simulink model "uz_9ph_pmsm_model"  (R2021a)
settings: Solver=FixedStepAuto  StartTime=0.0  StopTime=.5  RelTol=1e-3
PreLoadFcn:
  | uz_pmsm_model_init_parameter
values from neighbouring files (symbols this model uses):
  c = 2/9*cat(1,tl1,tl2,tl3,tl4,tl5,tl6,tl7,tl8,tl9)    [uz_pmsm_model_9ph_init_parameter.m]
  friction_coefficient = 0.001    [uz_pmsm_model_9ph_init_parameter.m]
  inertia = 0.001    [uz_pmsm_model_9ph_init_parameter.m]
  k_i_d = 1000    [uz_pmsm_model_9ph_init_parameter.m]
  k_p_d = 100    [uz_pmsm_model_9ph_init_parameter.m]
  k_p_q = 100    [uz_pmsm_model_9ph_init_parameter.m]
  L_d = 30e-3    (= 0.03)    [uz_pmsm_model_9ph_init_parameter.m]
  L_o1 = 0.01    [uz_pmsm_model_9ph_init_parameter.m]
  L_o2 = 0.01    [uz_pmsm_model_9ph_init_parameter.m]
  L_q = 50e-3    (= 0.05)    [uz_pmsm_model_9ph_init_parameter.m]
  L_x1 = 0.01    [uz_pmsm_model_9ph_init_parameter.m]
  L_x2 = 0.01    [uz_pmsm_model_9ph_init_parameter.m]
  L_y1 = 0.01    [uz_pmsm_model_9ph_init_parameter.m]
  L_y2 = 0.01    [uz_pmsm_model_9ph_init_parameter.m]
  L_zero = 0.01    [uz_pmsm_model_9ph_init_parameter.m]
  polepair = 5    [uz_pmsm_model_9ph_init_parameter.m]
  psi_pm = 0.05    [uz_pmsm_model_9ph_init_parameter.m]
  R_1 = 0.1    [uz_pmsm_model_9ph_init_parameter.m]
  static_friction_torque = 0.01    [uz_pmsm_model_9ph_init_parameter.m]
  ts = 1/1e6    (= 1e-06)    [uz_pmsm_model_9ph_init_parameter.m]
libraries: pid_lib x2
settings Model: DataTypeOverride=Off  Creator=ts  LastModifiedBy=valen
settings SolverCC: AlgebraicLoopSolver=TrustRegion  AutoInsertRateTranBlk=on
settings DataIOCC: LimitDataPoints=on  SaveOutput=off  SaveTime=off
settings OptimizationCC: BlockReduction=off  ConditionallyExecuteInputs=off  DefaultParameterBehavior=Inlined  LifeSpan=inf
settings DebuggingCC: AlgebraicLoopMsg=error  SingleTaskRateTransMsg=error  AllowSymbolicDim=off  StrictBusMsg=ErrorOnBusTreatedAsVector  SFUnexpectedBacktrackingDiag=warning  SFNoUnconditionalDefaultTransitionDiag=warning  SFExecutionAtInitializationDiag=none  SFMachineParentedDataDiag=warning  ArithmeticOperatorsInVariantConditions=warning
settings HardwareCC: ProdBitPerPointer=32  ProdBitPerSizeT=32  ProdBitPerPtrDiffT=32  ProdLargestAtomicFloat=None  ProdIntDivRoundTo=Undefined  ProdEndianess=Unspecified  ProdWordSize=32  ProdHWDeviceType=ASIC/FPGA->ASIC/FPGA  ProdEqTarget=off
settings SFSimCC: SimUseLocalCustomCode=off  CustomCodeUndefinedFunction=UseInterfaceOnly
settings RTWCC: RTWUseLocalCustomCode=off
settings CodeAppCC: StateflowObjectComments=on
settings GRTTargetCC: TargetLangStandard=C89/C90 (ANSI)
settings ConfigComp: CovScope=ReferencedModels  CovMetricSettings=dw  CovSaveCumulativeToWorkspaceVar=on  CovSaveSingleToWorkspaceVar=on  CovExternalEMLEnable=off  CovSFcnEnable=off

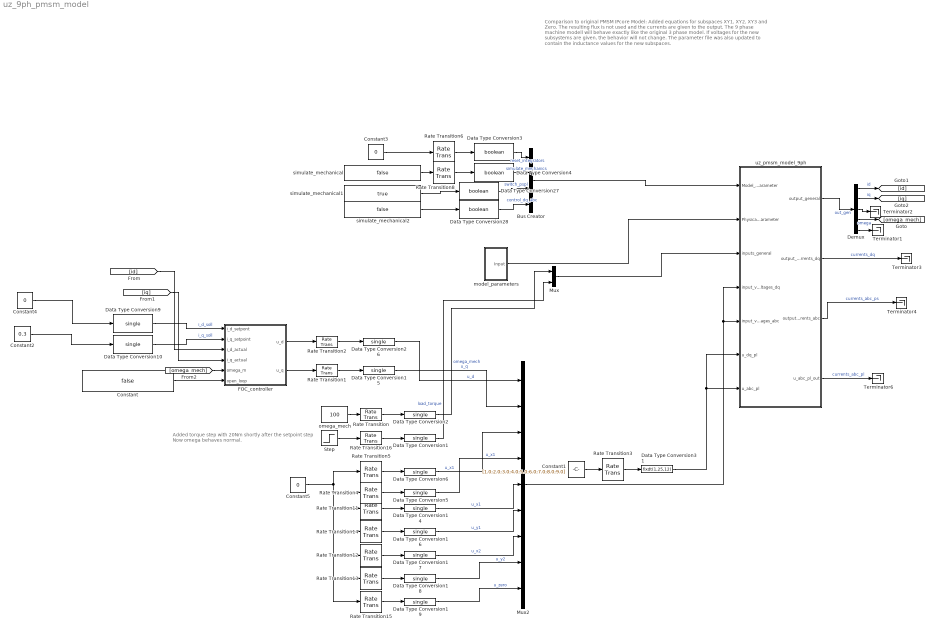
== system uz_9ph_pmsm_model ==
  note: Added torque step with 20Nm shortly after the setpoint step
      | Now omega behaves normal.
  note: Comparison to original PMSM IPcore Model:
      | Added equations for subspaces XY1, XY2, XY3 and Zero. The resulting flux is not used and the currents are given to the output.
      | The 9 phase machine modell will behave exactly like the original 3 phase model. If voltages for the new subsystems are given, the behavior will not change.
      | The parameter file was also updated to contain the inductance values for the new subspaces.
  Bus Creator : BusCreator  Inputs=4
  Constant : Constant  Value=false
  Constant1 : Constant  Value=[1.0;2.0;3.0;4.0;5.0;6.0;7.0;8.0;9.0]
  Constant2 : Constant  Value=0.3
  Constant3 : Constant  Value=0
  Constant4 : Constant  Value=0
  Constant5 : Constant  Value=0
  Data Type Conversion{1..2,5..6,14..19,26} (11 alike) : DataTypeConversion  OutDataTypeStr=single  RndMeth=Nearest
  Data Type Conversion10 : DataTypeConversion  OutDataTypeStr=single
  Data Type Conversion{3..4,27..28} (4 alike) : DataTypeConversion  OutDataTypeStr=boolean
  Data Type Conversion31 : DataTypeConversion  OutDataTypeStr=fixdt(1,25,12)  RndMeth=Nearest
  Data Type Conversion9 : DataTypeConversion  OutDataTypeStr=single
  Demux : Demux  Outputs=5
  FOC_controller : Subsystem
  Mux : Mux  Inputs=2
  Mux2 : Mux  Inputs=9
  Rate Transition{,1..6,8,11..16} (14 alike) : RateTransition  OutPortSampleTime=ts
  Step : Step  Time=0.25  After=20  SampleTime=0
  Terminator{1..4,6} (5 alike) : Terminator
  model_parameters : Subsystem
  omega_mech : Constant  Value=100
  simulate_mechanical : Constant  Value=false
  simulate_mechanical1 : Constant  Value=true
  simulate_mechanical2 : Constant  Value=false
  uz_pmsm_model_9ph : Subsystem  TreatAsAtomicUnit=on
  wires:
  Rate Transition/1 -> Data Type Conversion2/1
  Rate Transition1/1 -> Data Type Conversion15/1
  Rate Transition2/1 -> Data Type Conversion26/1
  Rate Transition6/1 -> Data Type Conversion3/1
  Constant3/1 -> Rate Transition6/1
  Rate Transition8/1 -> Data Type Conversion4/1
  simulate_mechanical/1 -> Rate Transition8/1
  Step/1 -> Rate Transition16/1
  Rate Transition16/1 -> Data Type Conversion1/1
  Constant4/1 -> Data Type Conversion9/1
  uz_pmsm_model_9ph/1(output_general) -> Demux/1  "out_gen"
  Data Type Conversion9/1 -> FOC_controller/1(i_d_setpont)  "i_d_soll"
  Data Type Conversion10/1 -> FOC_controller/2(i_q_setpoint)  "i_q_soll"
  FOC_controller/1(u_d) -> Rate Transition2/1
  FOC_controller/2(u_q) -> Rate Transition1/1
  omega_mech/1 -> Rate Transition/1
  Constant/1 -> FOC_controller/6(open_loop)
  Rate Transition11/1 -> Data Type Conversion14/1
  Data Type Conversion14/1 -> Mux2/5  "u_x1"
  Rate Transition13/1 -> Data Type Conversion18/1
  Rate Transition12/1 -> Data Type Conversion17/1
  Rate Transition14/1 -> Data Type Conversion16/1
  Data Type Conversion16/1 -> Mux2/6  "u_y1"
  Data Type Conversion17/1 -> Mux2/7  "u_x2"
  Data Type Conversion18/1 -> Mux2/8  "u_y2"
  Data Type Conversion19/1 -> Mux2/9  "u_zero"
  Rate Transition15/1 -> Data Type Conversion19/1
  Constant5/1 -> Rate Transition15/1, Rate Transition13/1, Rate Transition12/1, Rate Transition14/1, Rate Transition11/1, Rate Transition4/1, Rate Transition5/1
  model_parameters/1(Input) -> uz_pmsm_model_9ph/2(Physical_Parameter)
  Data Type Conversion4/1 -> Bus Creator/2  "simulate_mechanics"
  Data Type Conversion3/1 -> Bus Creator/1  "reset_integrators"
  Data Type Conversion27/1 -> Bus Creator/3  "switch_pspl"
  Data Type Conversion28/1 -> Bus Creator/4  "control_dq_abc"
  Bus Creator/1 -> uz_pmsm_model_9ph/1(Model_Parameter)
  uz_pmsm_model_9ph/2(output_currents_dq) -> Terminator3/1  "currents_dq"
  uz_pmsm_model_9ph/3(output_currents_abc) -> Terminator4/1  "currents_abc_ps"
  Mux2/1 -> uz_pmsm_model_9ph/5(input_voltages_abc), uz_pmsm_model_9ph/4(input_voltages_dq)
  Mux/1 -> uz_pmsm_model_9ph/3(inputs_general)
  Data Type Conversion2/1 -> Mux/1  "omega_mech"
  Data Type Conversion1/1 -> Mux/2  "load_torque"
  Constant1/1 -> Rate Transition3/1
  Rate Transition3/1 -> Data Type Conversion31/1
  Data Type Conversion31/1 -> uz_pmsm_model_9ph/7(u_abc_pl), uz_pmsm_model_9ph/6(u_dq_pl)
  uz_pmsm_model_9ph/4(u_abc_pl_out) -> Terminator6/1  "currents_abc_pl"
  simulate_mechanical1/1 -> Data Type Conversion27/1
  simulate_mechanical2/1 -> Data Type Conversion28/1
  [omega_mech] -> FOC_controller/5(omega_m)
  Demux/4 -> [omega_mech]  "omega"
  Demux/1 -> [id]  "id"
  Demux/2 -> [iq]  "iq"
  [iq] -> FOC_controller/4(i_q_actual)
  [id] -> FOC_controller/3(i_d_actual)
  Constant2/1 -> Data Type Conversion10/1
  Demux/5 -> Terminator1/1
  Demux/3 -> Terminator2/1
  Data Type Conversion26/1 -> Mux2/1  "u_d"
  Data Type Conversion15/1 -> Mux2/2  "u_q"
  Rate Transition4/1 -> Data Type Conversion5/1
  Rate Transition5/1 -> Data Type Conversion6/1
  Data Type Conversion6/1 -> Mux2/3  "u_x1"
  Data Type Conversion5/1 -> Mux2/4  "u_x1"

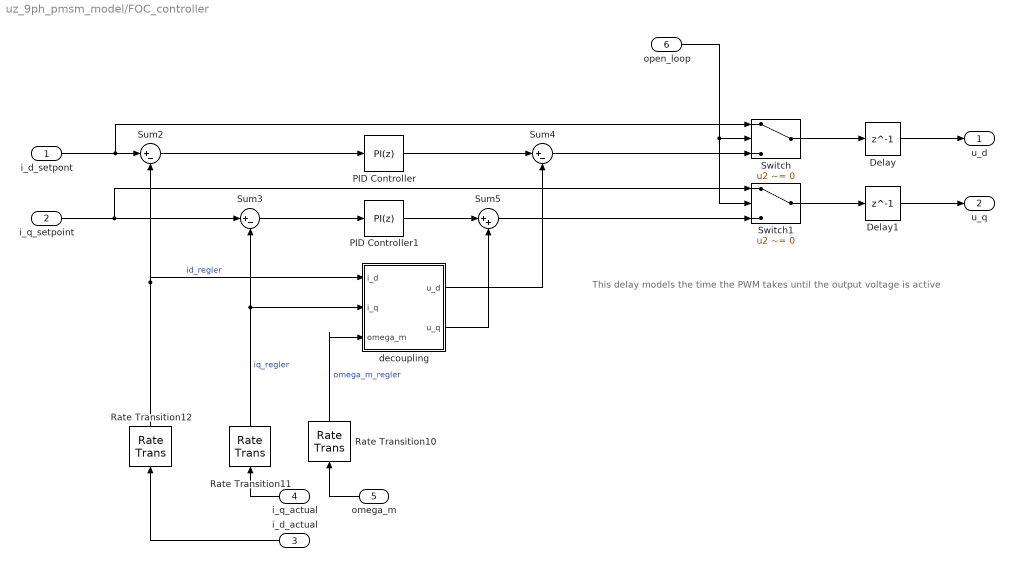
== system uz_9ph_pmsm_model/FOC_controller ==
  note: This delay models the time the PWM takes until the output voltage is active
  i_d_setpont : Inport
  i_q_setpoint : Inport  Port=2
  i_d_actual : Inport  Port=3
  i_q_actual : Inport  Port=4
  omega_m : Inport  Port=5
  open_loop : Inport  Port=6
  Delay : Delay  DelayLength=1
  Delay1 : Delay  DelayLength=1
  PID Controller : pid_lib/PID Controller  Controller=PI  Form=Parallel  TimeDomain=Discrete-time  UseExternalTs=off  SampleTime=-1  IntegratorMethod=Forward Euler  FilterMethod=Forward Euler  ControllerParametersSource=internal  P=k_p_d  I=k_i_d  D=0  UseFilter=on  N=100  TunerSelectOption=Transfer Function Based (PID Tuner App)  InitialConditionSource=internal  InitialConditionForIntegrator=0  InitialConditionForFilter=0  DifferentiatorICPrevScaledInput=0  ExternalReset=none  TrackingMode=off  Kt=1  LimitOutput=off  SatLimitsSource=internal  UpperSaturationLimit=inf  LowerSaturationLimit=-inf  LinearizeAsGain=on  AntiWindupMode=none  Kb=1  POutMin=[]  POutMax=[]  IOutMin=[]  IOutMax=[]  DOutMin=[]  DOutMax=[]  NOutMin=[]  NOutMax=[]  SumOutMin=[]  SumOutMax=[]  SaturationOutMin=[]  SaturationOutMax=[]  PParamMin=[]  PParamMax=[]  IParamMin=[]  IParamMax=[]  DParamMin=[]  DParamMax=[]  NParamMin=[]  NParamMax=[]  KbParamMin=[]  KbParamMax=[]  KtParamMin=[]  KtParamMax=[]  KbOutMin=[]  KbOutMax=[]  KtOutMin=[]  KtOutMax=[]  IntegratorOutMin=[]  IntegratorOutMax=[]  FilterOutMin=[]  FilterOutMax=[]  SumI1OutMin=[]  SumI1OutMax=[]  SumI2OutMin=[]  SumI2OutMax=[]  SumI3OutMin=[]  SumI3OutMax=[]  SumI4OutMin=[]  SumI4OutMax=[]  SumDOutMin=[]  SumDOutMax=[]  DifferentiatorOutMin=[]  DifferentiatorOutMax=[]  FilterDiffOutCoefMin=[]  FilterDiffOutCoefMax=[]  ReciprocalOutMin=[]  ReciprocalOutMax=[]  SumDenOutMin=[]  SumDenOutMax=[]  SumNumOutMin=[]  SumNumOutMax=[]  DivideOutMin=[]  DivideOutMax=[]  UdiffTsProdOutMin=[]  UdiffTsProdOutMax=[]  NTsProdOutMin=[]  NTsProdOutMax=[]  UintegralTsProdOutMin=[]  UintegralTsProdOutMax=[]  UngainTsProdOutMin=[]  UngainTsProdOutMax=[]  IntegratorContinuousStateAttributes=''  IntegratorStateMustResolveToSignalObject=off  IntegratorRTWStateStorageClass=Auto  FilterContinuousStateAttributes=''  FilterStateMustResolveToSignalObject=off  FilterRTWStateStorageClass=Auto  ParallelPVariant=InternalParameters  IdealPVariant=Disabled  IVariant=InternalParameters  DVariant=Disabled  IntegratorVariant=Discrete  SatVariant=Disabled  AWVariant=Passthrough  PCopyVariant=Disabled  TRVariant=Disabled  FdbkBlocksVariant=Forward  IdealPFdbkVariant=Disabled  SatFdbkVariant=Disabled  DerivativeFilterVariant=Disabled  NVariant=Disabled  NCopyVariant=Disabled_SignalSpec  FilterICVariant=Disabled  IntegratorICVariant=InternalICs  ExternalResetVariant=Disabled  TRSumVariant=Passthrough  SumFdbkVariant=Disabled  SumVariant=Sum_PI  TsampFilterVariant=InternalTs  TsampNgainVariant=Passthrough  TsampIntegralVariant=Passthrough  ExternalSaturationOutDataTypeStr=Inherit: Same as second input
  PID Controller1 : pid_lib/PID Controller  Controller=PI  Form=Parallel  TimeDomain=Discrete-time  UseExternalTs=off  SampleTime=-1  IntegratorMethod=Forward Euler  FilterMethod=Forward Euler  ControllerParametersSource=internal  P=k_p_q  I=k_i_d  D=0  UseFilter=on  N=100  TunerSelectOption=Transfer Function Based (PID Tuner App)  InitialConditionSource=internal  InitialConditionForIntegrator=0  InitialConditionForFilter=0  DifferentiatorICPrevScaledInput=0  ExternalReset=none  TrackingMode=off  Kt=1  LimitOutput=off  SatLimitsSource=internal  UpperSaturationLimit=inf  LowerSaturationLimit=-inf  LinearizeAsGain=on  AntiWindupMode=none  Kb=1  POutMin=[]  POutMax=[]  IOutMin=[]  IOutMax=[]  DOutMin=[]  DOutMax=[]  NOutMin=[]  NOutMax=[]  SumOutMin=[]  SumOutMax=[]  SaturationOutMin=[]  SaturationOutMax=[]  PParamMin=[]  PParamMax=[]  IParamMin=[]  IParamMax=[]  DParamMin=[]  DParamMax=[]  NParamMin=[]  NParamMax=[]  KbParamMin=[]  KbParamMax=[]  KtParamMin=[]  KtParamMax=[]  KbOutMin=[]  KbOutMax=[]  KtOutMin=[]  KtOutMax=[]  IntegratorOutMin=[]  IntegratorOutMax=[]  FilterOutMin=[]  FilterOutMax=[]  SumI1OutMin=[]  SumI1OutMax=[]  SumI2OutMin=[]  SumI2OutMax=[]  SumI3OutMin=[]  SumI3OutMax=[]  SumI4OutMin=[]  SumI4OutMax=[]  SumDOutMin=[]  SumDOutMax=[]  DifferentiatorOutMin=[]  DifferentiatorOutMax=[]  FilterDiffOutCoefMin=[]  FilterDiffOutCoefMax=[]  ReciprocalOutMin=[]  ReciprocalOutMax=[]  SumDenOutMin=[]  SumDenOutMax=[]  SumNumOutMin=[]  SumNumOutMax=[]  DivideOutMin=[]  DivideOutMax=[]  UdiffTsProdOutMin=[]  UdiffTsProdOutMax=[]  NTsProdOutMin=[]  NTsProdOutMax=[]  UintegralTsProdOutMin=[]  UintegralTsProdOutMax=[]  UngainTsProdOutMin=[]  UngainTsProdOutMax=[]  IntegratorContinuousStateAttributes=''  IntegratorStateMustResolveToSignalObject=off  IntegratorRTWStateStorageClass=Auto  FilterContinuousStateAttributes=''  FilterStateMustResolveToSignalObject=off  FilterRTWStateStorageClass=Auto  ParallelPVariant=InternalParameters  IdealPVariant=Disabled  IVariant=InternalParameters  DVariant=Disabled  IntegratorVariant=Discrete  SatVariant=Disabled  AWVariant=Passthrough  PCopyVariant=Disabled  TRVariant=Disabled  FdbkBlocksVariant=Forward  IdealPFdbkVariant=Disabled  SatFdbkVariant=Disabled  DerivativeFilterVariant=Disabled  NVariant=Disabled  NCopyVariant=Disabled_SignalSpec  FilterICVariant=Disabled  IntegratorICVariant=InternalICs  ExternalResetVariant=Disabled  TRSumVariant=Passthrough  SumFdbkVariant=Disabled  SumVariant=Sum_PI  TsampFilterVariant=InternalTs  TsampNgainVariant=Passthrough  TsampIntegralVariant=Passthrough  ExternalSaturationOutDataTypeStr=Inherit: Same as second input
  Rate Transition10 : RateTransition  OutPortSampleTime=ts_regler
  Rate Transition11 : RateTransition  OutPortSampleTime=ts_regler
  Rate Transition12 : RateTransition  OutPortSampleTime=ts_regler
  Sum2 : Sum  Inputs=|+-
  Sum3 : Sum  Inputs=|+-
  Sum4 : Sum  Inputs=|+-
  Sum5 : Sum  Inputs=|++
  Switch : Switch  Criteria=u2 ~= 0
  Switch1 : Switch  Criteria=u2 ~= 0
  decoupling : Subsystem
  u_d : Outport
  u_q : Outport  Port=2
  wires:
  PID Controller/1 -> Sum4/1
  PID Controller1/1 -> Sum5/1
  Sum4/1 -> Switch/3
  i_d_actual/1 -> Rate Transition12/1
  i_d_setpont/1 -> Switch/1, Sum2/1
  Sum2/1 -> PID Controller/1
  Sum5/1 -> Switch1/3
  omega_m/1 -> Rate Transition10/1
  Sum3/1 -> PID Controller1/1
  i_q_actual/1 -> Rate Transition11/1
  Rate Transition12/1 -> decoupling/1(i_d), Sum2/2  "id_regler"
  Rate Transition11/1 -> decoupling/2(i_q), Sum3/2  "iq_regler"
  i_q_setpoint/1 -> Switch1/1, Sum3/1
  open_loop/1 -> Switch1/2, Switch/2
  Rate Transition10/1 -> decoupling/3(omega_m)  "omega_m_regler"
  decoupling/1(u_d) -> Sum4/2
  decoupling/2(u_q) -> Sum5/2
  Switch/1 -> Delay/1
  Switch1/1 -> Delay1/1
  Delay/1 -> u_d/1
  Delay1/1 -> u_q/1

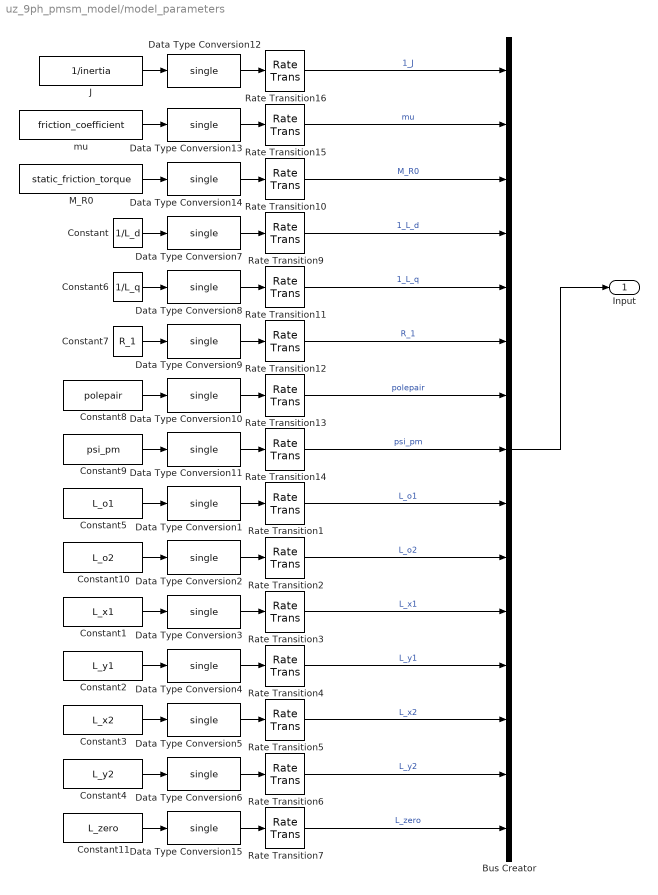
== system uz_9ph_pmsm_model/model_parameters ==
  Bus Creator : BusCreator  Inputs=15
  Constant : Constant  Value=1/L_d
  Constant1 : Constant  Value=L_x1
  Constant10 : Constant  Value=L_o2
  Constant11 : Constant  Value=L_zero
  Constant2 : Constant  Value=L_y1
  Constant3 : Constant  Value=L_x2
  Constant4 : Constant  Value=L_y2
  Constant5 : Constant  Value=L_o1
  Constant6 : Constant  Value=1/L_q
  Constant7 : Constant  Value=R_1
  Constant8 : Constant  Value=polepair
  Constant9 : Constant  Value=psi_pm
  Data Type Conversion{1..15} (15 alike) : DataTypeConversion  OutDataTypeStr=single
  J : Constant  Value=1/inertia
  M_R0 : Constant  Value=static_friction_torque
  Rate Transition{1..7,9..16} (15 alike) : RateTransition  OutPortSampleTime=ts
  mu : Constant  Value=friction_coefficient
  Input : Outport
  wires:
  Data Type Conversion12/1 -> Rate Transition16/1
  Data Type Conversion7/1 -> Rate Transition9/1
  Rate Transition10/1 -> Bus Creator/3  "M_R0"
  Rate Transition14/1 -> Bus Creator/8  "psi_pm"
  Data Type Conversion14/1 -> Rate Transition10/1
  Rate Transition12/1 -> Bus Creator/6  "R_1"
  Rate Transition16/1 -> Bus Creator/1  "1_J"
  Rate Transition13/1 -> Bus Creator/7  "polepair"
  Bus Creator/1 -> Input/1
  Data Type Conversion11/1 -> Rate Transition14/1
  Constant8/1 -> Data Type Conversion10/1
  Data Type Conversion9/1 -> Rate Transition12/1
  Rate Transition15/1 -> Bus Creator/2  "mu"
  Constant6/1 -> Data Type Conversion8/1
  Rate Transition9/1 -> Bus Creator/4  "1_L_d"
  J/1 -> Data Type Conversion12/1
  Data Type Conversion8/1 -> Rate Transition11/1
  Data Type Conversion10/1 -> Rate Transition13/1
  mu/1 -> Data Type Conversion13/1
  M_R0/1 -> Data Type Conversion14/1
  Rate Transition11/1 -> Bus Creator/5  "1_L_q"
  Data Type Conversion13/1 -> Rate Transition15/1
  Constant7/1 -> Data Type Conversion9/1
  Constant9/1 -> Data Type Conversion11/1
  Constant/1 -> Data Type Conversion7/1
  Data Type Conversion1/1 -> Rate Transition1/1
  Data Type Conversion2/1 -> Rate Transition2/1
  Data Type Conversion3/1 -> Rate Transition3/1
  Data Type Conversion4/1 -> Rate Transition4/1
  Data Type Conversion5/1 -> Rate Transition5/1
  Data Type Conversion6/1 -> Rate Transition6/1
  Constant11/1 -> Data Type Conversion15/1
  Data Type Conversion15/1 -> Rate Transition7/1
  Rate Transition1/1 -> Bus Creator/9  "L_o1"
  Rate Transition7/1 -> Bus Creator/15  "L_zero"
  Rate Transition6/1 -> Bus Creator/14  "L_y2"
  Rate Transition5/1 -> Bus Creator/13  "L_x2"
  Rate Transition4/1 -> Bus Creator/12  "L_y1"
  Rate Transition3/1 -> Bus Creator/11  "L_x1"
  Rate Transition2/1 -> Bus Creator/10  "L_o2"
  Constant4/1 -> Data Type Conversion6/1
  Constant3/1 -> Data Type Conversion5/1
  Constant2/1 -> Data Type Conversion4/1
  Constant1/1 -> Data Type Conversion3/1
  Constant5/1 -> Data Type Conversion1/1
  Constant10/1 -> Data Type Conversion2/1

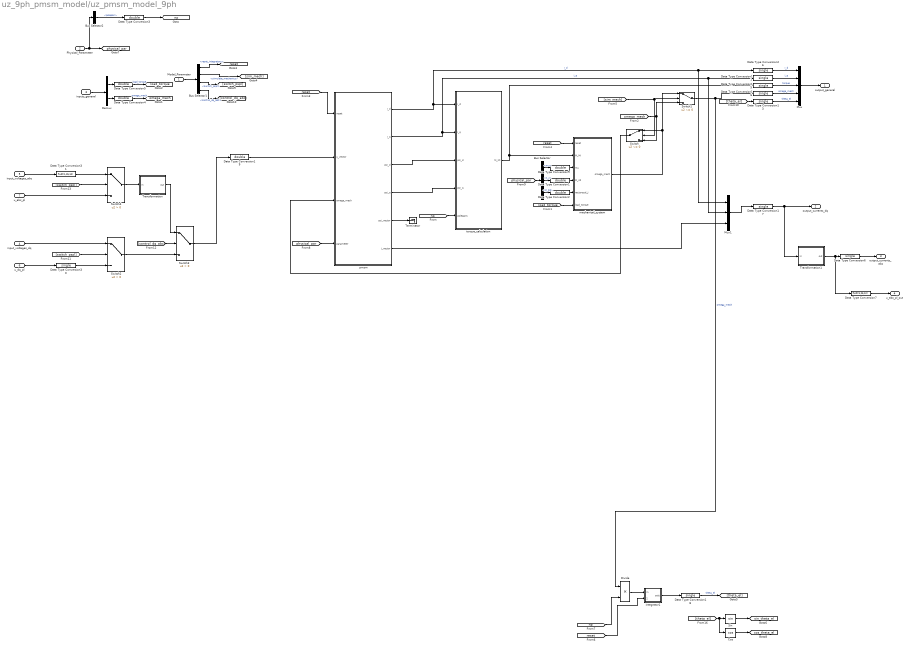
== system uz_9ph_pmsm_model/uz_pmsm_model_9ph ==
  Model_Parameter : Inport
  Physical_Parameter : Inport  Port=2
  inputs_general : Inport  Port=3
  input_voltages_dq : Inport  Port=4
  input_voltages_abc : Inport  Port=5
  u_dq_pl : Inport  Port=6
  u_abc_pl : Inport  Port=7
  Bus Selector : BusSelector  OutputSignals=mu,1_J,M_R0
  Bus Selector1 : BusSelector  OutputSignals=reset_integrators,simulate_mechanics,switch_pspl,control_dq_abc
  Bus Selector2 : BusSelector  OutputSignals=polepair
  Cos : Trigonometry  Operator=cos
  Data Type Conversion{1..5,9,19} (7 alike) : DataTypeConversion  OutDataTypeStr=double  RndMeth=Nearest
  Data Type Conversion{6,11,13,15..18,26,30} (9 alike) : DataTypeConversion  OutDataTypeStr=single  RndMeth=Nearest
  Data Type Conversion31 : DataTypeConversion  OutDataTypeStr=fixdt(1,25,12)  RndMeth=Nearest
  Data Type Conversion7 : DataTypeConversion  OutDataTypeStr=fixdt(1,25,12)  RndMeth=Nearest
  Demux : Demux  Outputs=2
  Divide : Product  Inputs=**
  Mux : Mux  Inputs=5
  Mux1 : Mux  Inputs=3
  Sin : Trigonometry
  Switch : Switch  Criteria=u2 ~= 0
  Switch1 : Switch  Criteria=u2 ~= 0
  Switch2 : Switch  Criteria=u2 > Threshold
  Switch3 : Switch  Criteria=u2 > Threshold
  Switch4 : Switch  Criteria=u2 > Threshold
  Terminator : Terminator
  Transformation : Subsystem
  Transformation1 : Subsystem
  integrator1 : Subsystem
  mechanical_system : Subsystem
  pmsm : Subsystem
  torque_calculation : Subsystem
  output_general : Outport
  output_currents_dq : Outport  Port=2
  output_currents_abc : Outport  Port=3
  u_abc_pl_out : Outport  Port=4
  tag scope: cos_theta_el=global, load_torque=global, np=global, omega_mech=global, physical_par=global, reset=global, sin_theta_el=global
  wires:
  Switch/1 -> pmsm/3(omega_mech)
  pmsm/3(psi_d) -> torque_calculation/3(psi_d)
  pmsm/4(psi_q) -> torque_calculation/4(psi_q)
  [sim_mech] -> Switch1/2, Switch/2
  torque_calculation/1(M_Mi) -> Data Type Conversion15/1, mechanical_system/2(M_Mi)
  mechanical_system/1(omega_mech) -> Switch/1, Switch1/1
  pmsm/2(I_q) -> Mux1/2, Data Type Conversion11/1, torque_calculation/2(I_q)  "i_q"
  pmsm/1(I_d) -> Mux1/1, Data Type Conversion26/1, torque_calculation/1(I_d)  "i_d"
  Data Type Conversion16/1 -> Mux/4  "omega_mech"
  Data Type Conversion15/1 -> Mux/3  "torque"
  Data Type Conversion11/1 -> Mux/2  "i_q"
  Data Type Conversion26/1 -> Mux/1  "i_d"
  inputs_general/1 -> Demux/1
  Mux/1 -> output_general/1
  [np] -> torque_calculation/5(polepairs)
  pmsm/5(psi_vector) -> Terminator/1
  Data Type Conversion4/1 -> [omega_mech]  "omega_mech"
  Data Type Conversion5/1 -> [load_torque]  "load_torque"
  [load_torque] -> mechanical_system/6(load_torque)
  [omega_mech] -> Switch/3, Switch1/3
  [reset] -> pmsm/1(reset)
  [reset] -> mechanical_system/1(reset)
  Model_Parameter/1 -> Bus Selector1/1
  Data Type Conversion13/1 -> Mux/5  "theta_el"
  input_voltages_dq/1 -> Switch2/1
  Bus Selector1/1 -> [reset]  "<reset_integrators>"
  Bus Selector1/2 -> [sim_mech]  "<simulate_mechanics>"
  Bus Selector1/3 -> [switch_pspl]  "<switch_pspl>"
  Bus Selector1/4 -> [control_dq_abc]  "<control_dq_abc>"
  input_voltages_abc/1 -> Data Type Conversion31/1
  Transformation1/1(out) -> Data Type Conversion7/1, Data Type Conversion6/1
  Data Type Conversion17/1 -> Transformation1/1(in), output_currents_dq/1
  Cos/1 -> [cos_theta_el]
  [theta_el] -> Cos/1, Sin/1
  integrator1/1(outt) -> Data Type Conversion18/1
  [reset] -> integrator1/2(reset)
  Data Type Conversion18/1 -> [theta_el]  "theta_el"
  Sin/1 -> [sin_theta_el]
  Divide/1 -> integrator1/1(in)
  Switch1/1 -> Divide/1, Data Type Conversion16/1  "omega_mech"
  [np] -> Divide/2
  u_dq_pl/1 -> Data Type Conversion30/1
  u_abc_pl/1 -> Switch4/3
  Data Type Conversion19/1 -> pmsm/2(u_vector)
  Physical_Parameter/1 -> Bus Selector2/1, [physical_par]
  [physical_par] -> pmsm/4(parameter)
  [physical_par] -> Bus Selector/1
  Data Type Conversion9/1 -> mechanical_system/3(mu)
  Data Type Conversion1/1 -> mechanical_system/4(M_n0)
  Data Type Conversion2/1 -> mechanical_system/5(reciprocal_J)
  Bus Selector/1 -> Data Type Conversion9/1  "<mu>"
  Bus Selector/2 -> Data Type Conversion1/1  "<1_J>"
  Bus Selector/3 -> Data Type Conversion2/1  "<M_R0>"
  Bus Selector2/1 -> Data Type Conversion3/1  "<polepair>"
  Data Type Conversion3/1 -> [np]
  Demux/2 -> Data Type Conversion4/1
  Demux/1 -> Data Type Conversion5/1
  [theta_el] -> Data Type Conversion13/1
  [switch_pspl] -> Switch2/2
  Data Type Conversion30/1 -> Switch2/3
  Switch2/1 -> Switch3/3
  [control_dq_abc] -> Switch3/2
  Switch3/1 -> Data Type Conversion19/1
  Data Type Conversion31/1 -> Switch4/1
  [switch_pspl] -> Switch4/2
  Switch4/1 -> Transformation/1(in)
  Transformation/1(out) -> Switch3/1
  pmsm/6(I_vector) -> Mux1/3
  Mux1/1 -> Data Type Conversion17/1
  Data Type Conversion6/1 -> output_currents_abc/1
  Data Type Conversion7/1 -> u_abc_pl_out/1

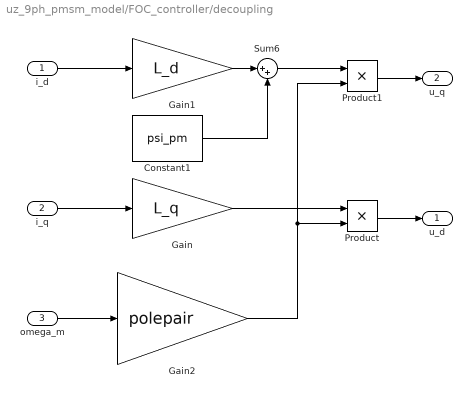
== system uz_9ph_pmsm_model/FOC_controller/decoupling ==
  i_d : Inport
  i_q : Inport  Port=2
  omega_m : Inport  Port=3
  Constant1 : Constant  Value=psi_pm  SampleTime=-1
  Gain : Gain  Gain=L_q
  Gain1 : Gain  Gain=L_d
  Gain2 : Gain  Gain=polepair
  Product : Product
  Product1 : Product
  Sum6 : Sum  Inputs=|++
  u_d : Outport
  u_q : Outport  Port=2
  wires:
  Gain/1 -> Product/1
  Gain2/1 -> Product1/2, Product/2
  Product1/1 -> u_q/1
  i_d/1 -> Gain1/1
  Product/1 -> u_d/1
  Gain1/1 -> Sum6/1
  i_q/1 -> Gain/1
  Constant1/1 -> Sum6/2
  Sum6/1 -> Product1/1
  omega_m/1 -> Gain2/1

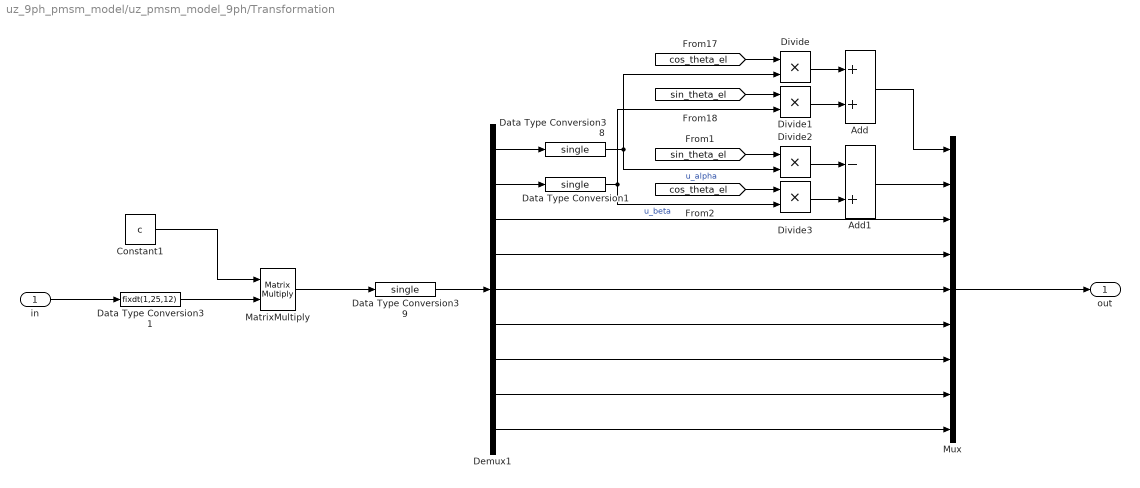
== system uz_9ph_pmsm_model/uz_pmsm_model_9ph/Transformation ==
  in : Inport
  Add : Sum
  Add1 : Sum  Inputs=-+
  Constant1 : Constant  Value=c  OutDataTypeStr=fixdt(1,18)  SampleTime=-1
  Data Type Conversion1 : DataTypeConversion  OutDataTypeStr=single  RndMeth=Nearest
  Data Type Conversion31 : DataTypeConversion  OutDataTypeStr=fixdt(1,25,12)  RndMeth=Nearest
  Data Type Conversion38 : DataTypeConversion  OutDataTypeStr=single  RndMeth=Nearest
  Data Type Conversion39 : DataTypeConversion  OutDataTypeStr=single  RndMeth=Nearest
  Demux1 : Demux  Outputs=9
  Divide{,1..3} (4 alike) : Product  Inputs=**
  MatrixMultiply : Product  Multiplication=Matrix(*)
  Mux : Mux  Inputs=9
  out : Outport
  wires:
  Demux1/3 -> Mux/3
  Demux1/4 -> Mux/4
  Demux1/5 -> Mux/5
  Demux1/6 -> Mux/6
  Demux1/7 -> Mux/7
  Demux1/8 -> Mux/8
  Demux1/9 -> Mux/9
  Mux/1 -> out/1
  Demux1/1 -> Data Type Conversion38/1
  Demux1/2 -> Data Type Conversion1/1
  Add1/1 -> Mux/2
  Add/1 -> Mux/1
  Data Type Conversion38/1 -> Divide/2, Divide2/2  "u_alpha"
  Data Type Conversion1/1 -> Divide1/2, Divide3/2  "u_beta"
  Divide/1 -> Add/1
  Divide1/1 -> Add/2
  [sin_theta_el] -> Divide1/1
  [cos_theta_el] -> Divide/1
  [sin_theta_el] -> Divide2/1
  [cos_theta_el] -> Divide3/1
  Divide3/1 -> Add1/2
  Divide2/1 -> Add1/1
  MatrixMultiply/1 -> Data Type Conversion39/1
  Constant1/1 -> MatrixMultiply/1
  Data Type Conversion39/1 -> Demux1/1
  in/1 -> Data Type Conversion31/1
  Data Type Conversion31/1 -> MatrixMultiply/2

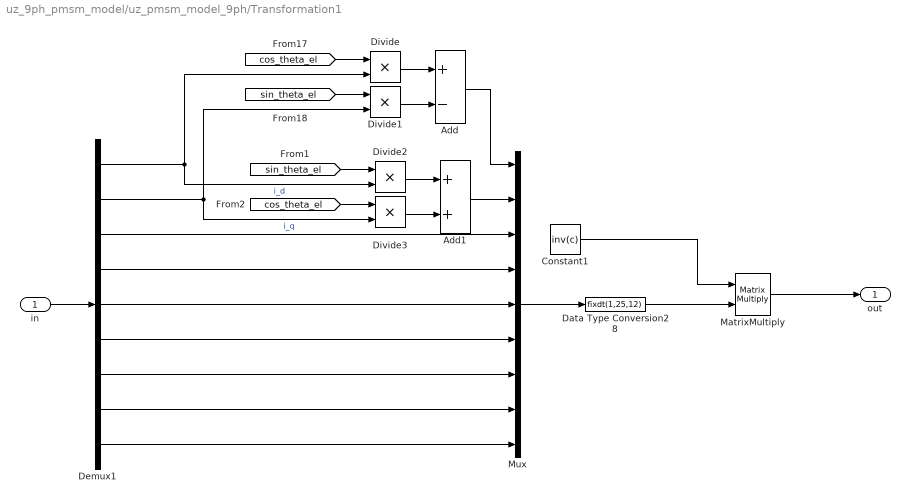
== system uz_9ph_pmsm_model/uz_pmsm_model_9ph/Transformation1 ==
  in : Inport
  Add : Sum  Inputs=+-
  Add1 : Sum
  Constant1 : Constant  Value=inv(c)  OutDataTypeStr=fixdt(1,18)  SampleTime=-1
  Data Type Conversion28 : DataTypeConversion  OutDataTypeStr=fixdt(1,25,12)  RndMeth=Nearest
  Demux1 : Demux  Outputs=9
  Divide{,1..3} (4 alike) : Product  Inputs=**
  MatrixMultiply : Product  Multiplication=Matrix(*)
  Mux : Mux  Inputs=9
  out : Outport
  wires:
  in/1 -> Demux1/1
  Mux/1 -> Data Type Conversion28/1
  Demux1/8 -> Mux/8
  Demux1/6 -> Mux/6
  Demux1/4 -> Mux/4
  Demux1/3 -> Mux/3
  Demux1/5 -> Mux/5
  Demux1/9 -> Mux/9
  Demux1/7 -> Mux/7
  [sin_theta_el] -> Divide1/1
  Demux1/2 -> Divide3/2, Divide1/2  "i_q"
  Add/1 -> Mux/1
  Divide/1 -> Add/1
  [cos_theta_el] -> Divide/1
  Divide1/1 -> Add/2
  Demux1/1 -> Divide2/2, Divide/2  "i_d"
  Divide3/1 -> Add1/2
  [sin_theta_el] -> Divide2/1
  Divide2/1 -> Add1/1
  [cos_theta_el] -> Divide3/1
  Add1/1 -> Mux/2
  Data Type Conversion28/1 -> MatrixMultiply/2
  Constant1/1 -> MatrixMultiply/1
  MatrixMultiply/1 -> out/1

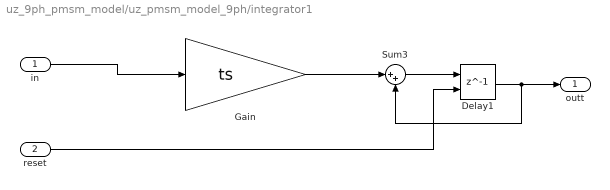
== system uz_9ph_pmsm_model/uz_pmsm_model_9ph/integrator1 ==
  in : Inport
  reset : Inport  Port=2
  Delay1 : Delay  DelayLength=1  ExternalReset=Level
      settings: InputPortMap=u0,r5
  Gain : Gain  Gain=ts  OutDataTypeStr=double
  Sum3 : Sum  Inputs=|++  OutDataTypeStr=double
  outt : Outport
  wires:
  Sum3/1 -> Delay1/1
  Delay1/1 -> outt/1, Sum3/2
  reset/1 -> Delay1/2
  Gain/1 -> Sum3/1
  in/1 -> Gain/1

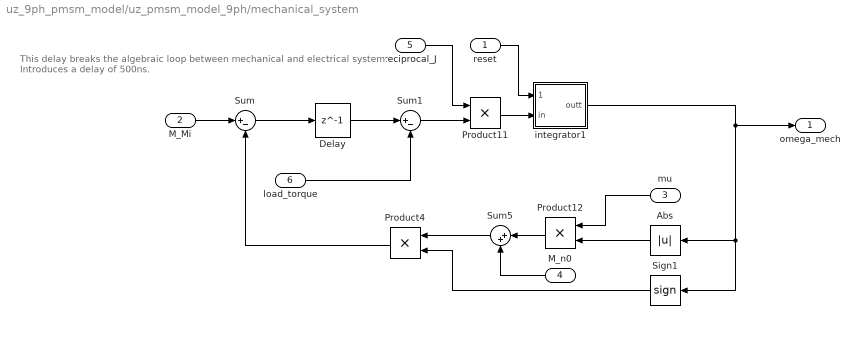
== system uz_9ph_pmsm_model/uz_pmsm_model_9ph/mechanical_system ==
  note: This delay breaks the algebraic loop between mechanical and electrical system.
      | Introduces a delay of 500ns.
  reset : Inport
  M_Mi : Inport  Port=2
  mu : Inport  Port=3
  M_n0 : Inport  Port=4
  reciprocal_J : Inport  Port=5
  load_torque : Inport  Port=6
  Abs : Abs
  Delay : Delay  DelayLength=1
  Product11 : Product
  Product12 : Product
  Product4 : Product
  Sign1 : Signum
  Sum : Sum  Inputs=|+-
  Sum1 : Sum  Inputs=|+-
  Sum5 : Sum  Inputs=|++
  integrator1 : Subsystem
  omega_mech : Outport
  wires:
  Product11/1 -> integrator1/2(in)
  Sum5/1 -> Product4/1
  Sign1/1 -> Product4/2
  integrator1/1(outt) -> Sign1/1, Abs/1, omega_mech/1
  Abs/1 -> Product12/2
  reset/1 -> integrator1/1(reset)
  Product12/1 -> Sum5/1
  mu/1 -> Product12/1
  M_n0/1 -> Sum5/2
  reciprocal_J/1 -> Product11/1
  M_Mi/1 -> Sum/1
  Sum1/1 -> Product11/2
  load_torque/1 -> Sum1/2
  Sum/1 -> Delay/1
  Product4/1 -> Sum/2
  Delay/1 -> Sum1/1

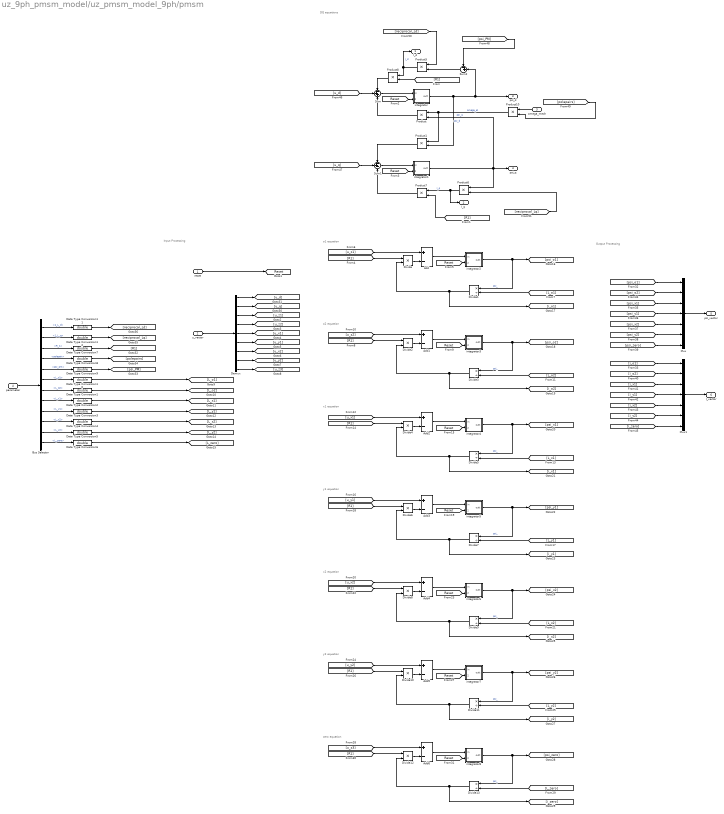
== system uz_9ph_pmsm_model/uz_pmsm_model_9ph/pmsm ==
  note: Input Processing
  note: o1 equation
  note: DQ equations
  note: o2 equation
  note: x1 equation
  note: y1 equation
  note: x2 equation
  note: y2 equation
  note: zero equation
  note: Output Processing
  reset : Inport
  u_vector : Inport  Port=2
  omega_mech : Inport  Port=3
  parameter : Inport  Port=4
  Add{,1..6} (7 alike) : Sum  Inputs=+-
  Bus Selector : BusSelector  OutputSignals=1_L_d,1_L_q,R_1,polepair,psi_pm,L_o1,L_o2,L_x1,L_y1,L_x2,L_y2,L_zero
  Data Type Conversion{1..12} (12 alike) : DataTypeConversion  OutDataTypeStr=double  RndMeth=Nearest
  Demux : Demux  Outputs=9
  Divide{,2,4,6,8,10,12} (7 alike) : Product  Inputs=**
  Divide{1,3,5,7,9,11,13} (7 alike) : Product  Inputs=*/
  Mux : Mux  Inputs=7
  Mux1 : Mux  Inputs=7
  Product{,1,5..8,10} (7 alike) : Product
  Sum : Sum  Inputs=-++
  Sum1 : Sum  Inputs=-+-
  Sum2 : Sum  Inputs=-+|
  integrator : Subsystem
  integrator1 : Subsystem
  integrator2 : Subsystem
  integrator3 : Subsystem
  integrator4 : Subsystem
  integrator5 : Subsystem
  integrator6 : Subsystem
  integrator7 : Subsystem
  integrator8 : Subsystem
  I_d : Outport
  I_q : Outport  Port=2
  psi_d : Outport  Port=3
  psi_q : Outport  Port=4
  psi_vector : Outport  Port=5
  I_vector : Outport  Port=6
  tag scope: Reset=global
  wires:
  omega_mech/1 -> Product10/1
  [u_q] -> Sum1/2
  Product/1 -> Sum/3
  Product5/1 -> I_d/1, Product8/1  "I_d"
  [reciprocal_Ld] -> Product5/1
  integrator1/1(outt) -> Product6/1, Product/2, psi_q/1  "psi_q"
  [u_d] -> Sum/2
  Product1/1 -> Sum1/1
  Sum/1 -> integrator/1(in)
  [psi_PM] -> Sum2/1
  Product6/1 -> I_q/1, Product7/1  "I_q"
  Product10/1 -> Product1/1, Product/1  "omega_el"
  integrator/1(outt) -> Product1/2, psi_d/1, Sum2/2  "psi_d"
  Sum2/1 -> Product5/2
  Product8/1 -> Sum/1
  [polepairs] -> Product10/2
  Product7/1 -> Sum1/3
  Sum1/1 -> integrator1/1(in)
  [R1] -> Product8/2
  [R1] -> Product7/2
  reset/1 -> [Reset]
  [Reset] -> integrator/2(reset)
  [Reset] -> integrator1/2(reset)
  u_vector/1 -> Demux/1
  [Reset] -> integrator2/2(reset)
  [L_o1] -> Divide1/2
  [u_z1] -> Add/1
  Divide1/1 -> [i_o1], Divide/2
  Divide/1 -> Add/2
  Add/1 -> integrator2/1(in)
  [R1] -> Divide/1
  integrator2/1(outt) -> [psi_o1], Divide1/1  "psi_"
  integrator3/1(outt) -> Divide3/1, [psi_o2]  "psi_"
  [R1] -> Divide2/1
  Add1/1 -> integrator3/1(in)
  Divide2/1 -> Add1/2
  Divide3/1 -> Divide2/2, [i_o2]
  [u_z2] -> Add1/1
  [L_o2] -> Divide3/2
  [Reset] -> integrator3/2(reset)
  [Reset] -> integrator4/2(reset)
  [L_x1] -> Divide5/2
  [u_x1] -> Add2/1
  Divide5/1 -> [i_x1], Divide4/2
  Divide4/1 -> Add2/2
  Add2/1 -> integrator4/1(in)
  [R1] -> Divide4/1
  integrator4/1(outt) -> [psi_x1], Divide5/1  "psi_"
  integrator5/1(outt) -> Divide7/1, [psi_y1]  "psi_"
  Add3/1 -> integrator5/1(in)
  Divide6/1 -> Add3/2
  Divide7/1 -> Divide6/2, [i_y1]
  [u_y1] -> Add3/1
  [L_y1] -> Divide7/2
  [Reset] -> integrator5/2(reset)
  [Reset] -> integrator6/2(reset)
  [L_x2] -> Divide9/2
  [u_x2] -> Add4/1
  Divide9/1 -> [i_x2], Divide8/2
  Divide8/1 -> Add4/2
  Add4/1 -> integrator6/1(in)
  [R1] -> Divide8/1
  integrator6/1(outt) -> [psi_x2], Divide9/1  "psi_"
  integrator7/1(outt) -> Divide11/1, [psi_y2]  "psi_"
  [R1] -> Divide10/1
  Add5/1 -> integrator7/1(in)
  Divide10/1 -> Add5/2
  Divide11/1 -> Divide10/2, [i_y2]
  [u_y2] -> Add5/1
  [L_y2] -> Divide11/2
  [Reset] -> integrator7/2(reset)
  [Reset] -> integrator8/2(reset)
  [L_zero] -> Divide13/2
  [u_z3] -> Add6/1
  Divide13/1 -> [i_zero], Divide12/2
  Divide12/1 -> Add6/2
  Add6/1 -> integrator8/1(in)
  [R1] -> Divide12/1
  integrator8/1(outt) -> [psi_zero], Divide13/1  "psi_"
  Mux/1 -> psi_vector/1
  Mux1/1 -> I_vector/1
  [psi_o1] -> Mux/1
  [i_o1] -> Mux1/1
  [psi_o2] -> Mux/2
  [psi_x1] -> Mux/3
  [psi_y1] -> Mux/4
  [psi_x2] -> Mux/5
  [psi_y2] -> Mux/6
  [psi_zero] -> Mux/7
  [i_o2] -> Mux1/2
  [i_x1] -> Mux1/3
  [i_y1] -> Mux1/4
  [i_x2] -> Mux1/5
  [i_y2] -> Mux1/6
  [i_zero] -> Mux1/7
  Demux/9 -> [u_z3]
  Demux/8 -> [u_y2]
  Demux/7 -> [u_x2]
  Demux/6 -> [u_y1]
  Demux/5 -> [u_x1]
  Demux/4 -> [u_z2]
  Demux/3 -> [u_z1]
  Demux/1 -> [u_d]
  Demux/2 -> [u_q]
  parameter/1 -> Bus Selector/1
  Bus Selector/12 -> Data Type Conversion6/1  "<L_zero>"
  Bus Selector/11 -> Data Type Conversion5/1  "<L_y2>"
  Bus Selector/10 -> Data Type Conversion4/1  "<L_x2>"
  Bus Selector/9 -> Data Type Conversion3/1  "<L_y1>"
  Bus Selector/8 -> Data Type Conversion2/1  "<L_x1>"
  Bus Selector/7 -> Data Type Conversion1/1  "<L_o2>"
  Bus Selector/6 -> Data Type Conversion10/1  "<L_o1>"
  Data Type Conversion10/1 -> [L_o1]
  Data Type Conversion1/1 -> [L_o2]
  Data Type Conversion2/1 -> [L_x1]
  Data Type Conversion3/1 -> [L_y1]
  Data Type Conversion4/1 -> [L_x2]
  Data Type Conversion5/1 -> [L_y2]
  Data Type Conversion6/1 -> [L_zero]
  Bus Selector/3 -> Data Type Conversion7/1  "<R_1>"
  Data Type Conversion7/1 -> [R1]
  Bus Selector/4 -> Data Type Conversion8/1  "<polepair>"
  Bus Selector/5 -> Data Type Conversion9/1  "<psi_pm>"
  Bus Selector/2 -> Data Type Conversion12/1  "<1_L_q>"
  Bus Selector/1 -> Data Type Conversion11/1  "<1_L_d>"
  Data Type Conversion8/1 -> [polepairs]
  Data Type Conversion9/1 -> [psi_PM]
  [reciprocal_Lq] -> Product6/2
  Data Type Conversion12/1 -> [reciprocal_Lq]
  Data Type Conversion11/1 -> [reciprocal_Ld]
  [R1] -> Divide6/1

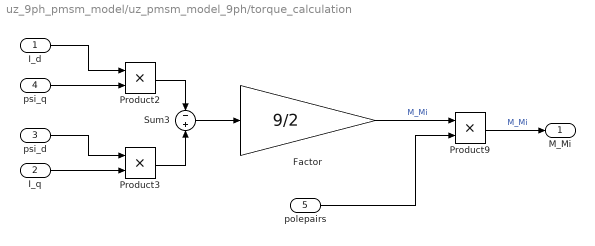
== system uz_9ph_pmsm_model/uz_pmsm_model_9ph/torque_calculation ==
  I_d : Inport
  I_q : Inport  Port=2
  psi_d : Inport  Port=3
  psi_q : Inport  Port=4
  polepairs : Inport  Port=5
  Factor : Gain  Gain=9/2
  Product2 : Product
  Product3 : Product
  Product9 : Product
  Sum3 : Sum  Inputs=-|+
  M_Mi : Outport
  wires:
  Sum3/1 -> Factor/1
  Product3/1 -> Sum3/2
  Product2/1 -> Sum3/1
  psi_q/1 -> Product2/2
  psi_d/1 -> Product3/1
  I_d/1 -> Product2/1
  I_q/1 -> Product3/2
  Product9/1 -> M_Mi/1  "M_Mi"
  polepairs/1 -> Product9/2
  Factor/1 -> Product9/1  "M_Mi"

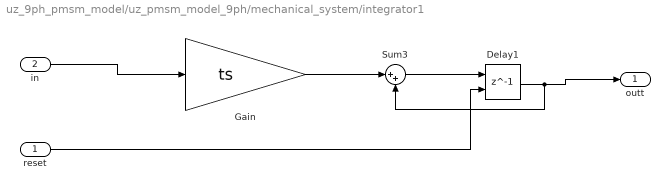
== system uz_9ph_pmsm_model/uz_pmsm_model_9ph/mechanical_system/integrator1 ==
  reset : Inport
  in : Inport  Port=2
  Delay1 : Delay  DelayLength=1  ExternalReset=Level
      settings: InputPortMap=u0,r5
  Gain : Gain  Gain=ts  OutDataTypeStr=double
  Sum3 : Sum  Inputs=|++  OutDataTypeStr=double
  outt : Outport
  wires:
  in/1 -> Gain/1
  Gain/1 -> Sum3/1
  reset/1 -> Delay1/2
  Sum3/1 -> Delay1/1
  Delay1/1 -> Sum3/2, outt/1

== system uz_9ph_pmsm_model/uz_pmsm_model_9ph/pmsm/integrator ==
  in : Inport
  reset : Inport  Port=2
  Delay1 : Delay  DelayLength=1  ExternalReset=Level
      settings: InputPortMap=u0,r5
  Gain : Gain  Gain=ts  OutDataTypeStr=double
  Sum3 : Sum  Inputs=|++  OutDataTypeStr=double
  outt : Outport
  wires:
  reset/1 -> Delay1/2
  Gain/1 -> Sum3/1
  in/1 -> Gain/1
  Delay1/1 -> outt/1, Sum3/2
  Sum3/1 -> Delay1/1

== system uz_9ph_pmsm_model/uz_pmsm_model_9ph/pmsm/integrator1 ==
  in : Inport
  reset : Inport  Port=2
  Delay1 : Delay  DelayLength=1  ExternalReset=Level
      settings: InputPortMap=u0,r5
  Gain : Gain  Gain=ts  OutDataTypeStr=double
  Sum3 : Sum  Inputs=|++  OutDataTypeStr=double
  outt : Outport
  wires:
  in/1 -> Gain/1
  Gain/1 -> Sum3/1
  reset/1 -> Delay1/2
  Delay1/1 -> Sum3/2, outt/1
  Sum3/1 -> Delay1/1

== system uz_9ph_pmsm_model/uz_pmsm_model_9ph/pmsm/integrator2 ==
  in : Inport
  reset : Inport  Port=2
  Delay1 : Delay  DelayLength=1  ExternalReset=Level
      settings: InputPortMap=u0,r5
  Gain : Gain  Gain=ts  OutDataTypeStr=double
  Sum3 : Sum  Inputs=|++  OutDataTypeStr=double
  outt : Outport
  wires:
  in/1 -> Gain/1
  Gain/1 -> Sum3/1
  reset/1 -> Delay1/2
  Delay1/1 -> Sum3/2, outt/1
  Sum3/1 -> Delay1/1

== system uz_9ph_pmsm_model/uz_pmsm_model_9ph/pmsm/integrator3 ==
  in : Inport
  reset : Inport  Port=2
  Delay1 : Delay  DelayLength=1  ExternalReset=Level
      settings: InputPortMap=u0,r5
  Gain : Gain  Gain=ts  OutDataTypeStr=double
  Sum3 : Sum  Inputs=|++  OutDataTypeStr=double
  outt : Outport
  wires:
  Sum3/1 -> Delay1/1
  Delay1/1 -> outt/1, Sum3/2
  reset/1 -> Delay1/2
  Gain/1 -> Sum3/1
  in/1 -> Gain/1

== system uz_9ph_pmsm_model/uz_pmsm_model_9ph/pmsm/integrator4 ==
  in : Inport
  reset : Inport  Port=2
  Delay1 : Delay  DelayLength=1  ExternalReset=Level
      settings: InputPortMap=u0,r5
  Gain : Gain  Gain=ts  OutDataTypeStr=double
  Sum3 : Sum  Inputs=|++  OutDataTypeStr=double
  outt : Outport
  wires:
  in/1 -> Gain/1
  Gain/1 -> Sum3/1
  reset/1 -> Delay1/2
  Delay1/1 -> Sum3/2, outt/1
  Sum3/1 -> Delay1/1

== system uz_9ph_pmsm_model/uz_pmsm_model_9ph/pmsm/integrator5 ==
  in : Inport
  reset : Inport  Port=2
  Delay1 : Delay  DelayLength=1  ExternalReset=Level
      settings: InputPortMap=u0,r5
  Gain : Gain  Gain=ts  OutDataTypeStr=double
  Sum3 : Sum  Inputs=|++  OutDataTypeStr=double
  outt : Outport
  wires:
  Sum3/1 -> Delay1/1
  Delay1/1 -> outt/1, Sum3/2
  reset/1 -> Delay1/2
  Gain/1 -> Sum3/1
  in/1 -> Gain/1

== system uz_9ph_pmsm_model/uz_pmsm_model_9ph/pmsm/integrator6 ==
  in : Inport
  reset : Inport  Port=2
  Delay1 : Delay  DelayLength=1  ExternalReset=Level
      settings: InputPortMap=u0,r5
  Gain : Gain  Gain=ts  OutDataTypeStr=double
  Sum3 : Sum  Inputs=|++  OutDataTypeStr=double
  outt : Outport
  wires:
  in/1 -> Gain/1
  Gain/1 -> Sum3/1
  reset/1 -> Delay1/2
  Delay1/1 -> Sum3/2, outt/1
  Sum3/1 -> Delay1/1

== system uz_9ph_pmsm_model/uz_pmsm_model_9ph/pmsm/integrator7 ==
  in : Inport
  reset : Inport  Port=2
  Delay1 : Delay  DelayLength=1  ExternalReset=Level
      settings: InputPortMap=u0,r5
  Gain : Gain  Gain=ts  OutDataTypeStr=double
  Sum3 : Sum  Inputs=|++  OutDataTypeStr=double
  outt : Outport
  wires:
  Sum3/1 -> Delay1/1
  Delay1/1 -> outt/1, Sum3/2
  reset/1 -> Delay1/2
  Gain/1 -> Sum3/1
  in/1 -> Gain/1

== system uz_9ph_pmsm_model/uz_pmsm_model_9ph/pmsm/integrator8 ==
  in : Inport
  reset : Inport  Port=2
  Delay1 : Delay  DelayLength=1  ExternalReset=Level
      settings: InputPortMap=u0,r5
  Gain : Gain  Gain=ts  OutDataTypeStr=double
  Sum3 : Sum  Inputs=|++  OutDataTypeStr=double
  outt : Outport
  wires:
  in/1 -> Gain/1
  Gain/1 -> Sum3/1
  reset/1 -> Delay1/2
  Delay1/1 -> Sum3/2, outt/1
  Sum3/1 -> Delay1/1
